simulink model "TRN_BRIDGE"  (R2021b)
settings: Solver=FixedStepAuto  StartTime=0.0  StopTime=10.0  RelTol=1e-3
settings Model: Creator=ascl  LastModifiedBy=sblee
settings SolverCC: AlgebraicLoopSolver=TrustRegion
settings DataIOCC: ReturnWorkspaceOutputs=off
settings OptimizationCC: DefaultParameterBehavior=Inlined  UseDivisionForNetSlopeComputation=on  GainParamInheritBuiltInType=on  UseFloatMulNetSlope=on  EnhancedBackFolding=on  PassReuseOutputArgsThreshold=0  OptimizeBlockOrder=speed  DifferentSizesBufferReuse=on  OptimizationCustomize=off
settings DebuggingCC: ParameterTunabilityLossMsg=error  SFMachineParentedDataDiag=warning  ArithmeticOperatorsInVariantConditions=warning
settings HardwareCC: TargetBitPerPointer=64  TargetBitPerSizeT=64  TargetBitPerPtrDiffT=64  TargetLongLongMode=on  TargetIntDivRoundTo=Zero  TargetEndianess=LittleEndian  TargetWordSize=64  TargetHWDeviceType=MATLAB Host  ProdEqTarget=off
settings SFSimCC: SimUseLocalCustomCode=off  MATLABDynamicMemAlloc=off  CustomCodeUndefinedFunction=UseInterfaceOnly
settings RTWCC: Description=Rapid Simulation Target  SystemTargetFile=rsim.tlc  TemplateMakefile=rsim_default_tmf  GenerateReport=on  RTWUseLocalCustomCode=off  LaunchReport=on
settings CodeAppCC: ForceParamTrailComments=on  OperatorAnnotations=on
settings RSimTargetCC: TargetLangStandard=C99 (ISO)

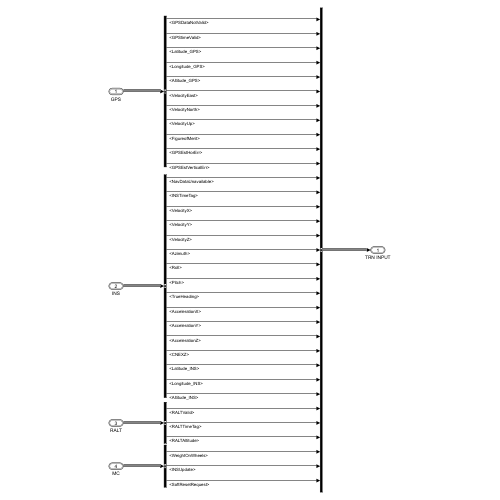
[thumbnail: Simulink's stored preview of the top-level diagram]
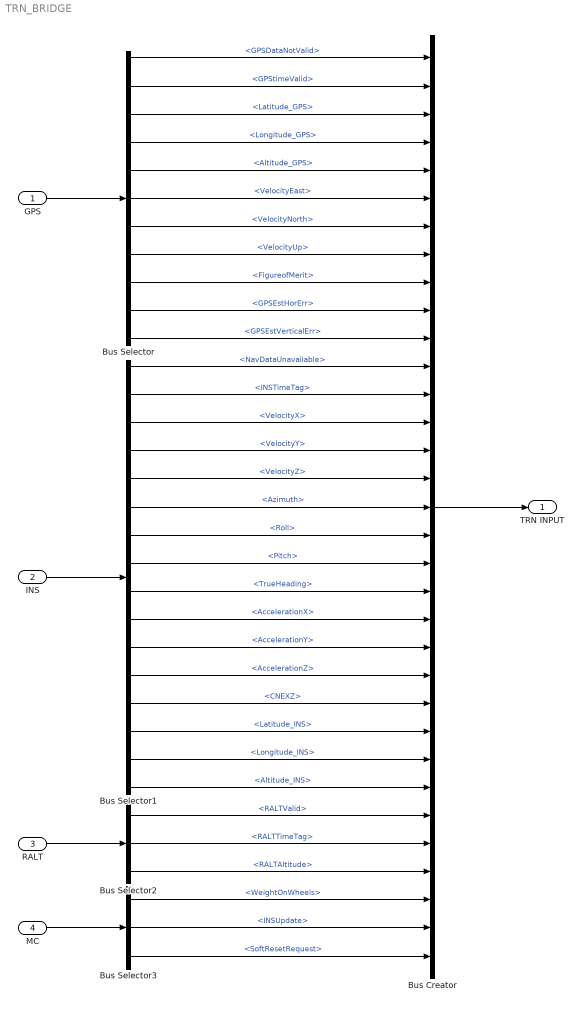
== system TRN_BRIDGE ==
  GPS : Inport  OutDataTypeStr=Bus: TRN_GPS
  INS : Inport  Port=2  OutDataTypeStr=Bus: TRN_INS
  RALT : Inport  Port=3  OutDataTypeStr=Bus: TRN_RALT
  MC : Inport  Port=4  OutDataTypeStr=Bus: TRN_MC
  Bus Creator : BusCreator  Inputs=33  OutDataTypeStr=Bus: TRNInput
  Bus Selector : BusSelector  OutputSignals=GPSDataNotValid,GPStimeValid,Latitude_GPS,Longitude_GPS,Altitude_GPS,VelocityEast,VelocityNorth,VelocityUp,FigureofMerit,GPSEstHorErr,GPSEstVerticalErr
  Bus Selector1 : BusSelector  OutputSignals=NavDataUnavailable,INSTimeTag,VelocityX,VelocityY,VelocityZ,Azimuth,Roll,Pitch,TrueHeading,AccelerationX,AccelerationY,AccelerationZ,CNEXZ,Latitude_INS,Longitude_INS,Altitude_INS
  Bus Selector2 : BusSelector  OutputSignals=RALTValid,RALTTimeTag,RALTAltitude
  Bus Selector3 : BusSelector  OutputSignals=WeightOnWheels,INSUpdate,SoftResetRequest
  TRN INPUT : Outport  OutDataTypeStr=Bus: TRNInput  VectorParamsAs1DForOutWhenUnconnected=off
  wires:
  INS/1 -> Bus Selector1/1
  GPS/1 -> Bus Selector/1
  RALT/1 -> Bus Selector2/1
  MC/1 -> Bus Selector3/1
  Bus Creator/1 -> TRN INPUT/1
  Bus Selector/2 -> Bus Creator/2  "<GPStimeValid>"
  Bus Selector/3 -> Bus Creator/3  "<Latitude_GPS>"
  Bus Selector/4 -> Bus Creator/4  "<Longitude_GPS>"
  Bus Selector/5 -> Bus Creator/5  "<Altitude_GPS>"
  Bus Selector/6 -> Bus Creator/6  "<VelocityEast>"
  Bus Selector/7 -> Bus Creator/7  "<VelocityNorth>"
  Bus Selector/8 -> Bus Creator/8  "<VelocityUp>"
  Bus Selector/9 -> Bus Creator/9  "<FigureofMerit>"
  Bus Selector/10 -> Bus Creator/10  "<GPSEstHorErr>"
  Bus Selector/11 -> Bus Creator/11  "<GPSEstVerticalErr>"
  Bus Selector2/2 -> Bus Creator/29  "<RALTTimeTag>"
  Bus Selector2/1 -> Bus Creator/28  "<RALTValid>"
  Bus Selector2/3 -> Bus Creator/30  "<RALTAltitude>"
  Bus Selector3/1 -> Bus Creator/31  "<WeightOnWheels>"
  Bus Selector3/2 -> Bus Creator/32  "<INSUpdate>"
  Bus Selector3/3 -> Bus Creator/33  "<SoftResetRequest>"
  Bus Selector1/1 -> Bus Creator/12  "<NavDataUnavailable>"
  Bus Selector1/2 -> Bus Creator/13  "<INSTimeTag>"
  Bus Selector1/3 -> Bus Creator/14  "<VelocityX>"
  Bus Selector1/4 -> Bus Creator/15  "<VelocityY>"
  Bus Selector1/5 -> Bus Creator/16  "<VelocityZ>"
  Bus Selector1/6 -> Bus Creator/17  "<Azimuth>"
  Bus Selector1/7 -> Bus Creator/18  "<Roll>"
  Bus Selector1/8 -> Bus Creator/19  "<Pitch>"
  Bus Selector1/9 -> Bus Creator/20  "<TrueHeading>"
  Bus Selector1/10 -> Bus Creator/21  "<AccelerationX>"
  Bus Selector1/11 -> Bus Creator/22  "<AccelerationY>"
  Bus Selector1/12 -> Bus Creator/23  "<AccelerationZ>"
  Bus Selector1/13 -> Bus Creator/24  "<CNEXZ>"
  Bus Selector1/14 -> Bus Creator/25  "<Latitude_INS>"
  Bus Selector1/15 -> Bus Creator/26  "<Longitude_INS>"
  Bus Selector1/16 -> Bus Creator/27  "<Altitude_INS>"
  Bus Selector/1 -> Bus Creator/1  "<GPSDataNotValid>"
